simulink model "mfunction2"  (Simulink 7.9)
settings: Solver=ode3  StartTime=0.0  StopTime=10.0  RelTol=1e-3
settings Model: Creator=ryusei  LastModifiedBy=ryusei
settings RTWCC: GenCodeOnly=on

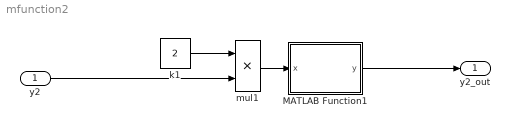
== system mfunction2 ==
  y2 : Inport
  MATLAB Function1 : MATLAB Function  TreatAsAtomicUnit=on
  k1 : Constant  Value=2
  mul1 : Product  RndMeth=Zero
  y2_out : Outport
  wires:
  k1/1 -> mul1/1
  y2/1 -> mul1/2
  mul1/1 -> MATLAB Function1/1(x)
  MATLAB Function1/1(y) -> y2_out/1

== matlab function MATLAB Function1 ==
  data: x input double; y output double
function y = fcn(x)
%#codegen
if x<0.5
    %y=1/sqrt(2);
    y=1
elseif x<=1
    %y=sqrt(2*x*(1-x));
    y=2
else
    y=0;
end

end
